simulink model "miss_03_v2"  (R2024a)
settings: Solver=ode4  StartTime=0.0  StopTime=100  FixedStep=0.01  RelTol=1e-3
settings Model: Creator=kg53848  LastModifiedBy=kg53848

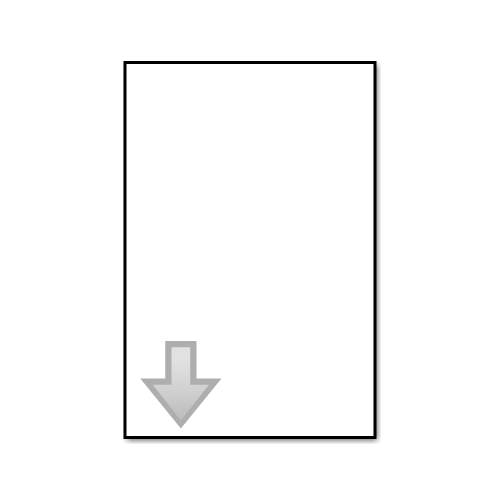
[thumbnail: Simulink's stored preview of the top-level diagram]
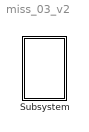
== system miss_03_v2 ==
  Subsystem : Subsystem  mask{fi=180, m=10, l=3, k=1, g=10}
      mask prompts: fi "wprowadz kat"; m "wprowadz mase"; l "wprowadz dlugosc"; k "wprowadz wsp tlumienia"; g "wprowadz przysp ziemskie"

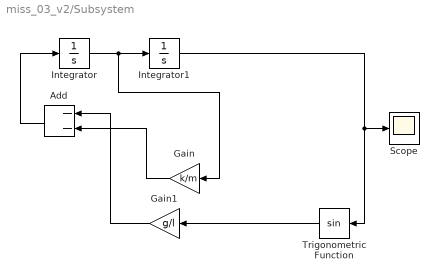
== system miss_03_v2/Subsystem ==
  Add : Sum  Inputs=--
  Gain : Gain  Gain=k/m
  Gain1 : Gain  Gain=g/l
  Integrator : Integrator
  Integrator1 : Integrator  InitialCondition=fi*pi/180
  Scope : Scope
  Trigonometric Function : Trigonometry
  wires:
  Integrator/1 -> Gain/1, Integrator1/1
  Gain/1 -> Add/2
  Integrator1/1 -> Scope/1, Trigonometric Function/1
  Gain1/1 -> Add/1
  Add/1 -> Integrator/1
  Trigonometric Function/1 -> Gain1/1
